simulink model "clik_second_order_inverse_2018"  (R2018b)
settings: Solver=VariableStepAuto  StartTime=0.0  StopTime=4  RelTol=1e-3
values from neighbouring files (symbols this model uses):
  q0 = [-0.927293431585 -1.28700579042 1 2.21429922201]    [kinematic_traj.mat]
  q0_dot = [0 0 0 0]    [kinematic_traj.mat]
  Tc = 0.001    [kinematic_traj.mat]
undefined symbols (not defined in the file or in its folder): DiscIntNeverNeededParam
settings Model: Creator=weichen  LastModifiedBy=15945

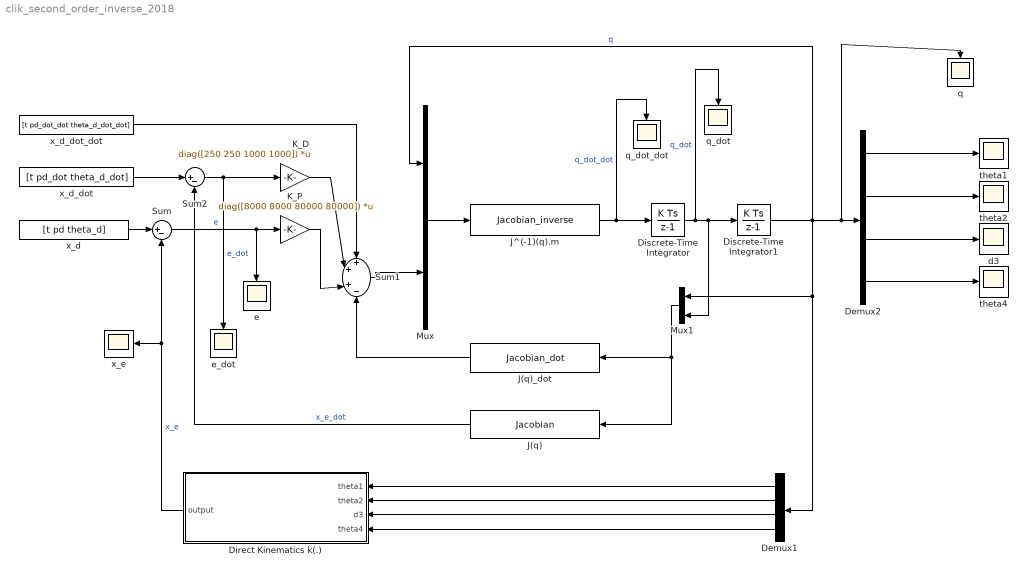
== system clik_second_order_inverse_2018 ==
  Demux1 : Demux
  Demux2 : Demux
  Direct Kinematics k(.) : MATLAB Function  TreatAsAtomicUnit=on
  Discrete-Time Integrator : DiscreteIntegrator  gainval=1  InitialCondition=q0_dot  SampleTime=Tc  ICPrevOutput=DiscIntNeverNeededParam  ICPrevScaledInput=DiscIntNeverNeededParam
  Discrete-Time Integrator1 : DiscreteIntegrator  InitialCondition=q0  SampleTime=Tc  ICPrevOutput=DiscIntNeverNeededParam  ICPrevScaledInput=DiscIntNeverNeededParam
  J(q) : MATLABFcn  MATLABFcn=Jacobian
  J(q)_dot : MATLABFcn  MATLABFcn=Jacobian_dot
  J^(-1)(q).m : MATLABFcn  MATLABFcn=Jacobian_inverse
  K_D : Gain  Gain=diag([250 250 1000 1000])  Multiplication=Matrix(K*u)
  K_P : Gain  Gain=diag([8000 8000 80000 80000])  Multiplication=Matrix(K*u)
  Mux : Mux  Inputs=2
  Mux1 : Mux  Inputs=2
  Sum : Sum  Inputs=|+-
  Sum1 : Sum  Inputs=+++-
  Sum2 : Sum  Inputs=|+-
  d3 : Scope
  e : Scope
  e_dot : Scope
  q : Scope
  q_dot : Scope
  q_dot_dot : Scope
  theta1 : Scope
  theta2 : Scope
  theta4 : Scope
  x_d : FromWorkspace  VariableName=[t pd theta_d]  SampleTime=Tc
  x_d_dot : FromWorkspace  VariableName=[t pd_dot theta_d_dot]  SampleTime=Tc
  x_d_dot_dot : FromWorkspace  VariableName=[t pd_dot_dot theta_d_dot_dot]  SampleTime=Tc
  x_e : Scope
  wires:
  x_d/1 -> Sum/1
  Direct Kinematics k(.)/1(output) -> Sum/2, x_e/1  "x_e"
  Sum/1 -> K_P/1, e/1  "e"
  K_P/1 -> Sum1/3
  J^(-1)(q).m/1 -> q_dot_dot/1, Discrete-Time Integrator/1  "q_dot_dot"
  Mux/1 -> J^(-1)(q).m/1
  Sum1/1 -> Mux/2
  Discrete-Time Integrator/1 -> Mux1/2, Discrete-Time Integrator1/1, q_dot/1  "q_dot"
  Demux1/1 -> Direct Kinematics k(.)/1(theta1)
  Demux1/2 -> Direct Kinematics k(.)/2(theta2)
  Demux1/3 -> Direct Kinematics k(.)/3(d3)
  Demux1/4 -> Direct Kinematics k(.)/4(theta4)
  Demux2/1 -> theta1/1
  Demux2/2 -> theta2/1
  Demux2/3 -> d3/1
  Demux2/4 -> theta4/1
  x_d_dot_dot/1 -> Sum1/1
  Discrete-Time Integrator1/1 -> Demux2/1, q/1, Demux1/1, Mux1/1, Mux/1  "q"
  x_d_dot/1 -> Sum2/1
  Sum2/1 -> e_dot/1, K_D/1  "e_dot"
  K_D/1 -> Sum1/2
  Mux1/1 -> J(q)/1, J(q)_dot/1
  J(q)/1 -> Sum2/2  "x_e_dot"
  J(q)_dot/1 -> Sum1/4

== matlab function clik_second_order_inverse_2018/Direct Kinematics k(.) ==
  data: theta1 input; output output; theta2 input; d3 input; theta4 input
function output = direct_kin(theta1,theta2,d3,theta4)
% Direct kinematics function of SCARA 
    A01 = [cos(theta1) -sin(theta1) 0 0.5.*cos(theta1);
           sin(theta1) cos(theta1) 0 0.5.*sin(theta1);
           0 0 1 0;
           0 0 0 1];
    A12 = [cos(theta2) -sin(theta2) 0 0.5.*cos(theta2);
           sin(theta2) cos(theta2) 0 0.5.*sin(theta2);
           0 0 1 0;
           0 0 0 1];
    A23 = [1 0 0 0;
           0 1 0 0;
           0 0 1 1-d3;
           0 0 0 1];
    A34 = [cos(theta4) -sin(theta4) 0 0;
           sin(theta4) cos(theta4) 0 0;
           0 0 1 0;
           0 0 0 1];
    A04 = A01*A12*A23*A34;
    P = [0.5*cos(theta1)+0.5*cos(theta1+theta2);0.5*sin(theta1)+0.5*sin(theta1+theta2);1-d3;(theta1+theta2+theta4)];
    output = P;
end
